simulink model "ex1_model"  (R2022b)
settings: Solver=FixedStepAuto  StartTime=0.0  StopTime=10.0  RelTol=1e-3
model workspace (MAT data in the model file):
  Kd = Simulink.Parameter
  Kd.Value = 100
  Kd.DataType = 'auto'
  Kd.Complexity = 'real'
  Kd.Dimensions = [1 1]
  Kp = Simulink.Parameter
  Kp.Value = 0.1
  Kp.DataType = 'auto'
  Kp.Complexity = 'real'
  Kp.Dimensions = [1 1]
  b = Simulink.Parameter
  b.Value = 100
  b.DataType = 'auto'
  b.Complexity = 'real'
  b.Dimensions = [1 1]
  k = Simulink.Parameter
  k.Value = 100
  k.DataType = 'auto'
  k.Complexity = 'real'
  k.Dimensions = [1 1]
  m = Simulink.Parameter
  m.Value = 1
  m.DataType = 'auto'
  m.Complexity = 'real'
  m.Dimensions = [1 1]
settings Model: Creator=erfuu  LastModifiedBy=erfuu
settings OptimizationCC: OptimizeBlockIOStorage=off  OptimizeDataStoreBuffers=off  BusAssignmentInplaceUpdate=off
settings DebuggingCC: SFUnexpectedBacktrackingDiag=warning  SFNoUnconditionalDefaultTransitionDiag=warning
settings RTWCC: GenerateReport=on  BuildConfiguration=Debug  LaunchReport=on
settings CodeAppCC: ForceParamTrailComments=on  MATLABSourceComments=on  EnableCustomComments=on
settings GRTTargetCC: CombineSignalStateStructs=on  SupportVariableSizeSignals=on  MultiInstanceErrorCode=Warning

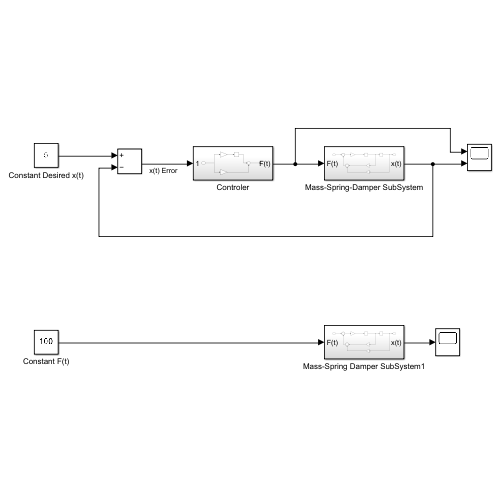
[thumbnail: Simulink's stored preview of the top-level diagram]
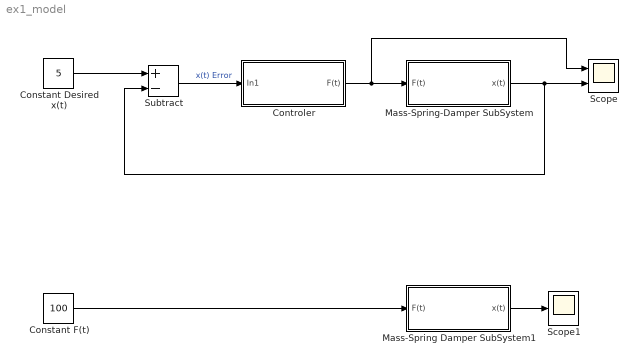
== system ex1_model ==
  Constant Desired x(t) : Constant  Value=5
  Constant F(t) : Constant  Value=100
  Controler : Subsystem
  Mass-Spring Damper SubSystem1 : Subsystem
  Mass-Spring-Damper SubSystem : Subsystem
  Scope : Scope  NumInputPorts=2
  Scope1 : Scope
  Subtract : Sum  Inputs=+-
  wires:
  Mass-Spring-Damper SubSystem/1(x(t)) -> Scope/2, Subtract/2
  Constant Desired x(t)/1 -> Subtract/1
  Subtract/1 -> Controler/1(In1)  "x(t) Error"
  Controler/1(F(t)) -> Mass-Spring-Damper SubSystem/1(F(t)), Scope/1
  Mass-Spring Damper SubSystem1/1(x(t)) -> Scope1/1
  Constant F(t)/1 -> Mass-Spring Damper SubSystem1/1(F(t))

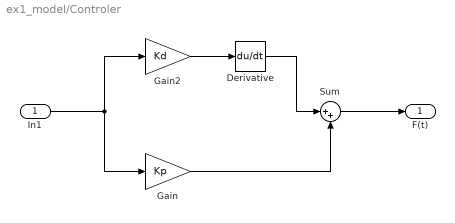
== system ex1_model/Controler ==
  In1 : Inport
  Derivative : Derivative
  Gain : Gain  Gain=Kp
  Gain2 : Gain  Gain=Kd
  Sum : Sum  Inputs=|++
  F(t) : Outport
  wires:
  In1/1 -> Gain2/1, Gain/1
  Gain2/1 -> Derivative/1
  Derivative/1 -> Sum/1
  Sum/1 -> F(t)/1
  Gain/1 -> Sum/2

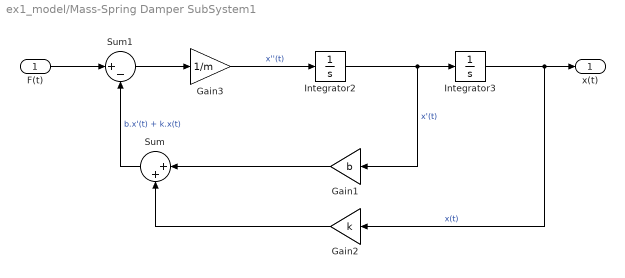
== system ex1_model/Mass-Spring Damper SubSystem1 ==
  F(t) : Inport
  Gain1 : Gain  Gain=b
  Gain2 : Gain  Gain=k
  Gain3 : Gain  Gain=1/m
  Integrator2 : Integrator
  Integrator3 : Integrator
  Sum : Sum  Inputs=|++
  Sum1 : Sum  Inputs=|+-
  x(t) : Outport
  wires:
  Integrator2/1 -> Integrator3/1, Gain1/1  "x'(t)"
  Integrator3/1 -> x(t)/1, Gain2/1  "x(t)"
  Gain3/1 -> Integrator2/1  "x''(t)"
  Gain2/1 -> Sum/2
  Gain1/1 -> Sum/1
  F(t)/1 -> Sum1/1
  Sum1/1 -> Gain3/1
  Sum/1 -> Sum1/2  "b.x'(t) + k.x(t)"

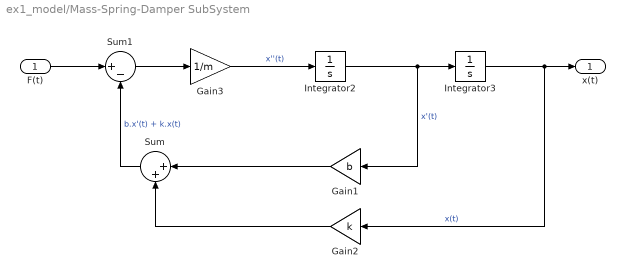
== system ex1_model/Mass-Spring-Damper SubSystem ==
  F(t) : Inport
  Gain1 : Gain  Gain=b
  Gain2 : Gain  Gain=k
  Gain3 : Gain  Gain=1/m
  Integrator2 : Integrator
  Integrator3 : Integrator
  Sum : Sum  Inputs=|++
  Sum1 : Sum  Inputs=|+-
  x(t) : Outport
  wires:
  Integrator2/1 -> Integrator3/1, Gain1/1  "x'(t)"
  Integrator3/1 -> x(t)/1, Gain2/1  "x(t)"
  Gain3/1 -> Integrator2/1  "x''(t)"
  Gain2/1 -> Sum/2
  Gain1/1 -> Sum/1
  F(t)/1 -> Sum1/1
  Sum1/1 -> Gain3/1
  Sum/1 -> Sum1/2  "b.x'(t) + k.x(t)"
